simulink model "RASscheme"  (R2020b)
settings: Solver=VariableStepAuto  StartTime=0.0  StopTime=10.0  RelTol=1e-3
settings Model: Creator=Tommaso  LastModifiedBy=Tommaso

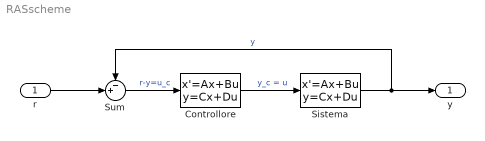
== system RASscheme ==
  r : Inport
  Controllore : StateSpace  InitialCondition=0
  Sistema : StateSpace  InitialCondition=0
  Sum : Sum  Inputs=-+|
  y : Outport
  wires:
  Controllore/1 -> Sistema/1  "y_c = u"
  Sistema/1 -> Sum/1, y/1  "y"
  Sum/1 -> Controllore/1  "r-y=u_c"
  r/1 -> Sum/2
